simulink model "Ebike_FaultModel"  (R2024b)
settings: Solver=VariableStepAuto  StartTime=0.0  StopTime=10.0  RelTol=1e-3  EnableMultiTasking=on
settings Model: Creator=s.maatoug  LastModifiedBy=s.maatoug
settings DebuggingCC: InheritedTsInSrcMsg=none

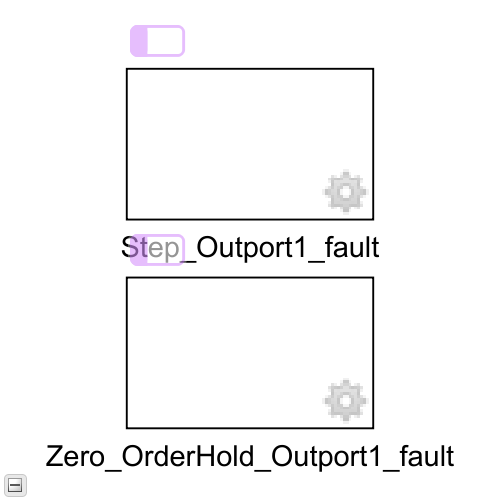
[thumbnail: Simulink's stored preview of the top-level diagram]
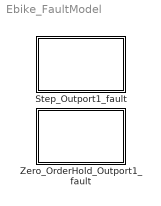
== system Ebike_FaultModel ==
  Step_Outport1_fault : Subsystem  TreatAsAtomicUnit=on  ScheduleAs=Aperiodic partition  PartitionName=PartitionFor_Step_Outport1_fault_423_000244  IsInjectorSS=on
  Zero_OrderHold_Outport1_fault : Subsystem  TreatAsAtomicUnit=on  ScheduleAs=Aperiodic partition  PartitionName=PartitionFor_Zero_OrderHold_Outport1_fault_434_001099  IsInjectorSS=on

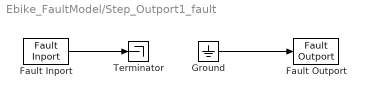
== system Ebike_FaultModel/Step_Outport1_fault ==
  Fault Inport : FaultInport
  Fault Outport : FaultOutport
  Ground : Ground
  Terminator : Terminator
  wires:
  Ground/1 -> Fault Outport/1
  Fault Inport/1 -> Terminator/1

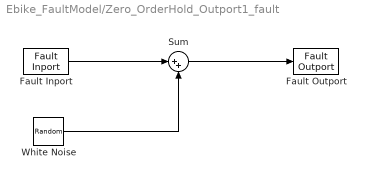
== system Ebike_FaultModel/Zero_OrderHold_Outport1_fault ==
  Fault Inport : FaultInport
  Fault Outport : FaultOutport
  Sum : Sum  Inputs=|++  OutDataTypeStr=Inherit: Inherit via back propagation
  White Noise : RandomNumber  DisableCoverage=on  Seed=[23341]
  wires:
  White Noise/1 -> Sum/2
  Sum/1 -> Fault Outport/1
  Fault Inport/1 -> Sum/1
